simulink model "MinimumJerkPlanner"  (R2024b)
settings: configuration reference "MCConfiguration" (kept outside this file)
undefined symbols (not defined in the file): acc_max, bVelocityMove, InitTrajectory, p0, pos_max, pos_min, target_pos, target_vel, Trajectory_set_pos_end, Trajectory_set_pos_raw, Trajectory_velocity_stop, Ts, vA, vel_max, velAvg, vInvT, vK0, vK1, vK2, vT, vTimer, vV, vX, xA, xInvT, xK0, xK1, xK2, xK3, xStar, xT, xTimer, xV, xX
libraries: simulink x6
settings Model: DataDictionary=MotionController.sldd  Creator=rpumpo  LastModifiedBy=mfussi
settings ConfigSetRef: SourceName=MCConfiguration

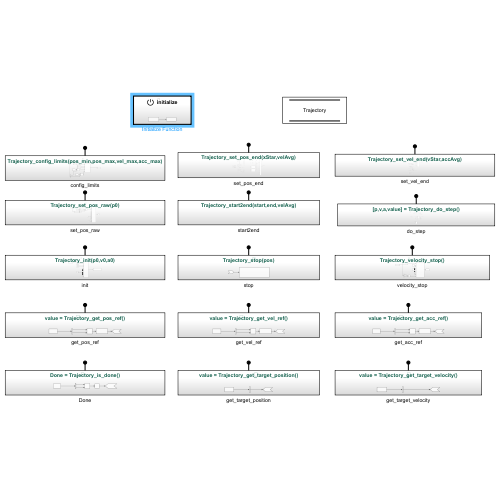
[thumbnail: Simulink's stored preview of the top-level diagram]
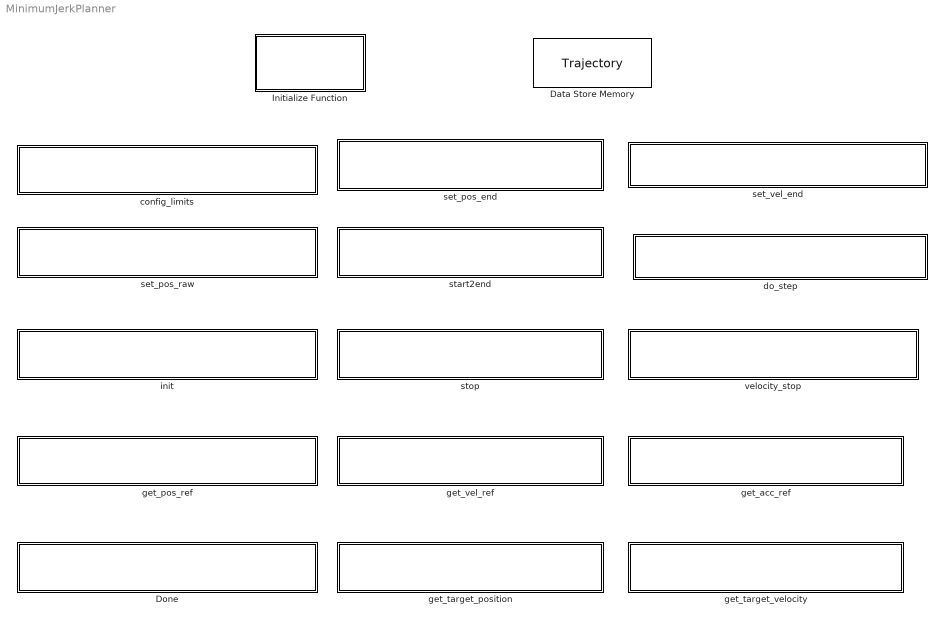
== system MinimumJerkPlanner ==
  Data Store Memory : DataStoreMemory  DataStoreName=Trajectory  WriteAfterWriteMsg=warning  ShowAdditionalParam=off  OutDataTypeStr=Bus: trajectoryhidParameters
  Done : Subsystem  TreatAsAtomicUnit=on
  Initialize Function : Subsystem  TreatAsAtomicUnit=on
  config_limits : Subsystem  TreatAsAtomicUnit=on
  do_step : Subsystem  TreatAsAtomicUnit=on
  get_acc_ref : Subsystem  TreatAsAtomicUnit=on
  get_pos_ref : Subsystem  TreatAsAtomicUnit=on
  get_target_position : Subsystem  TreatAsAtomicUnit=on
  get_target_velocity : Subsystem  TreatAsAtomicUnit=on
  get_vel_ref : Subsystem  TreatAsAtomicUnit=on
  init : Subsystem  TreatAsAtomicUnit=on
  set_pos_end : Subsystem  TreatAsAtomicUnit=on
  set_pos_raw : Subsystem  TreatAsAtomicUnit=on
  set_vel_end : Subsystem  TreatAsAtomicUnit=on
  start2end : Subsystem  TreatAsAtomicUnit=on
  stop : Subsystem  TreatAsAtomicUnit=on
  velocity_stop : Subsystem  TreatAsAtomicUnit=on

== system MinimumJerkPlanner/Done ==
  Trajectory_is_done : TriggerPort  TriggerType=function-call  IsSimulinkFunction=on  FunctionName=Trajectory_is_done  FunctionVisibility=scoped  VariantControl=(inherit)
  Add : Sum  Inputs=+-
  Bus Selector : BusSelector  OutputSignals=xTimer,xT
  Compare To Constant : simulink/Logic and Bit Operations/Compare To Constant  relop=>=  const=0  OutDataTypeStr=boolean
  Data Store Read : DataStoreRead  DataStoreName=Trajectory  IndexOptions=Index vector (dialog)  Indices=1  OutputSizes=1
  Done : ArgOut  OutDataTypeStr=boolean  ArgumentName=Done
  wires:
  Data Store Read/1 -> Bus Selector/1
  Bus Selector/2 -> Add/2  "<xT>"
  Bus Selector/1 -> Add/1  "<xTimer>"
  Add/1 -> Compare To Constant/1
  Compare To Constant/1 -> Done/1

== system MinimumJerkPlanner/Initialize Function ==
  Constant : Constant  Value=InitTrajectory  OutDataTypeStr=Bus: trajectoryhidParameters
  Data Store Write : DataStoreWrite  DataStoreName=Trajectory  IndexOptions=Index vector (dialog)  Indices=1  OutputSizes=1
  Event Listener : EventListener  DisableCoverage=on  EventName=reset
  wires:
  Constant/1 -> Data Store Write/1

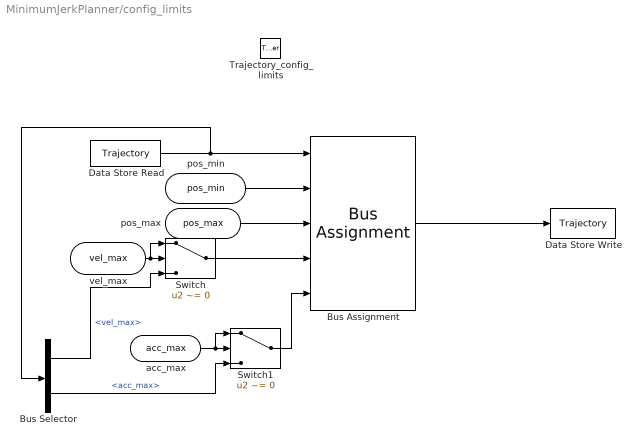
== system MinimumJerkPlanner/config_limits ==
  Trajectory_config_limits : TriggerPort  TriggerType=function-call  IsSimulinkFunction=on  FunctionName=Trajectory_config_limits  FunctionVisibility=scoped  VariantControl=(inherit)
  Bus Assignment : BusAssignment  AssignedSignals=pos_min,pos_max,vel_max,acc_max
  Bus Selector : BusSelector  OutputSignals=vel_max,acc_max
  Data Store Read : DataStoreRead  DataStoreName=Trajectory  IndexOptions=Index vector (dialog)  Indices=1  OutputSizes=1
  Data Store Write : DataStoreWrite  DataStoreName=Trajectory  IndexOptions=Index vector (dialog)  Indices=1  OutputSizes=1
  Switch : Switch  Criteria=u2 ~= 0  SaturateOnIntegerOverflow=off  InputSameDT=off
  Switch1 : Switch  Criteria=u2 ~= 0  SaturateOnIntegerOverflow=off  InputSameDT=off
  pos_min : ArgIn  OutDataTypeStr=single  ArgumentName=pos_min
  pos_max : ArgIn  Port=2  OutDataTypeStr=single  ArgumentName=pos_max
  vel_max : ArgIn  Port=3  OutDataTypeStr=single  ArgumentName=vel_max
  acc_max : ArgIn  Port=4  OutDataTypeStr=single  ArgumentName=acc_max
  wires:
  Data Store Read/1 -> Bus Selector/1, Bus Assignment/1
  pos_min/1 -> Bus Assignment/2
  pos_max/1 -> Bus Assignment/3
  Bus Assignment/1 -> Data Store Write/1
  vel_max/1 -> Switch/1, Switch/2
  Bus Selector/1 -> Switch/3  "<vel_max>"
  Switch/1 -> Bus Assignment/4
  acc_max/1 -> Switch1/1, Switch1/2
  Bus Selector/2 -> Switch1/3  "<acc_max>"
  Switch1/1 -> Bus Assignment/5

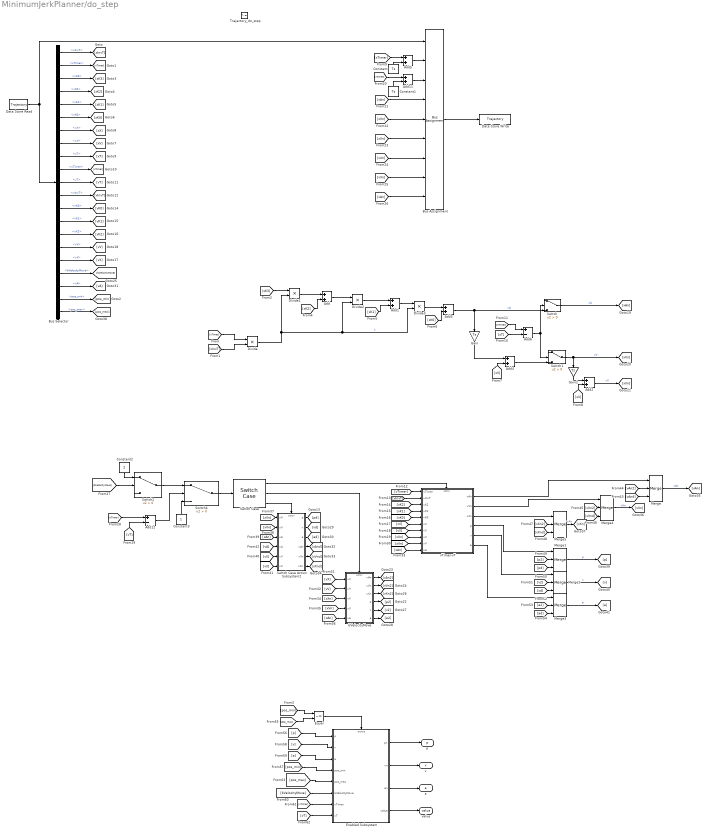
== system MinimumJerkPlanner/do_step ==
  Trajectory_do_step : TriggerPort  TriggerType=function-call  IsSimulinkFunction=on  FunctionName=Trajectory_do_step  FunctionVisibility=scoped  VariantControl=(inherit)
  Add{,1..5,11} (7 alike) : Sum
  Add12 : Sum  Inputs=+-
  Add6 : Sum  Inputs=+-
  Bus Assignment : BusAssignment  AssignedSignals=xTimer,vTimer,xA,xV,xX,vX,vV,vA
  Bus Selector : BusSelector  OutputSignals=xInvT,xTimer,xK3,xK2,xK1,xK0,xX,xV,xT,vTimer,vT,vInvT,vK0,vK1,vK2,vV,vX,bVelocityMove,vA,pos_min,pos_max
  Constant : Constant  Value=Ts  OutDataTypeStr=single
  Constant1 : Constant  Value=Ts  OutDataTypeStr=single
  Constant2 : Constant  Value=2
  Constant3 : Constant
  Data Store Read : DataStoreRead  DataStoreName=Trajectory  IndexOptions=Index vector (dialog)  Indices=1  OutputSizes=1
  Data Store Write : DataStoreWrite  DataStoreName=Trajectory  IndexOptions=Index vector (dialog)  Indices=1  OutputSizes=1
  Divide{,1..3} (4 alike) : Product  Inputs=**
  Enabled Subsystem : Subsystem  TreatAsAtomicUnit=on
  Equal : RelationalOperator  Operator=~=  OutDataTypeStr=boolean  RndMeth=Simplest  InputSameDT=off
  Gain : Gain  Gain=Ts
  Gain2 : Gain  Gain=Ts
  Merge{,1..5} (6 alike) : Merge  Inputs=3
  Switch{,1..2,4} (4 alike) : Switch  Criteria=u2 > Threshold  SaturateOnIntegerOverflow=off  InputSameDT=off
  Switch Case : SwitchCase  CaseConditions={1,2}
  Switch Case Action Subsystem2 : Subsystem  TreatAsAtomicUnit=on
  bVelocityMove : Subsystem  TreatAsAtomicUnit=on
  vTimer-vT : Subsystem  TreatAsAtomicUnit=on
  p : ArgOut  DisableCoverage=on  OutDataTypeStr=single  ArgumentName=p
  v : ArgOut  DisableCoverage=on  Port=2  OutDataTypeStr=single  ArgumentName=v
  a : ArgOut  DisableCoverage=on  Port=3  OutDataTypeStr=single  ArgumentName=a
  value : ArgOut  DisableCoverage=on  Port=4  OutDataTypeStr=int32  ArgumentName=value
  wires:
  Data Store Read/1 -> Bus Assignment/1, Bus Selector/1
  Add4/1 -> Switch1/3
  Add3/1 -> Switch/3, Gain/1  "xA"
  Bus Selector/1 -> [xInvT]  "<xInvT>"
  Bus Selector/2 -> [xTimer]  "<xTimer>"
  [xTimer] -> Divide/1
  [xInvT] -> Divide/2
  Divide/1 -> Divide1/2, Divide2/2, Divide3/2  "t"
  Bus Selector/3 -> [xK3]  "<xK3>"
  Bus Selector/4 -> [xK2]  "<xK2>"
  Bus Selector/5 -> [xK1]  "<xK1>"
  Bus Selector/6 -> [xK0]  "<xK0>"
  [xK3] -> Divide1/1
  Divide1/1 -> Add/1
  [xK2] -> Add/2
  Add/1 -> Divide2/1
  Divide2/1 -> Add1/1
  [xK1] -> Add1/2
  Add1/1 -> Divide3/1
  Divide3/1 -> Add3/1
  [xK0] -> Add3/2
  Bus Selector/7 -> [xX]  "<xX>"
  Bus Selector/8 -> [xV]  "<xV>"
  Gain/1 -> Add4/1
  [xV] -> Add4/2
  Gain2/1 -> Add2/1
  [xX] -> Add2/2
  [xTimer] -> Add5/1
  Constant/1 -> Add5/2
  Add5/1 -> Bus Assignment/2
  Bus Assignment/1 -> Data Store Write/1
  Bus Selector/9 -> [xT]  "<xT>"
  [xTimer] -> Add6/1
  [xT] -> Add6/2
  Add6/1 -> Switch/2, Switch1/2
  Switch1/1 -> Gain2/1, [xVn]  "xV"
  Bus Selector/10 -> [vTimer]  "<vTimer>"
  Bus Selector/11 -> [vT]  "<vT>"
  Bus Selector/12 -> [vInvT]  "<vInvT>"
  Bus Selector/13 -> [vK0]  "<vK0>"
  Bus Selector/14 -> [vK1]  "<vK1>"
  Bus Selector/15 -> [vK2]  "<vK2>"
  Bus Selector/16 -> [vV]  "<vV>"
  Bus Selector/17 -> [vX]  "<vX>"
  Switch/1 -> [xAn]  "xA"
  Add2/1 -> [xXn]  "xX"
  [xAn] -> Bus Assignment/4
  [xVn] -> Bus Assignment/5
  [xXn] -> Bus Assignment/6
  [vXn] -> Bus Assignment/7
  [vVn] -> Bus Assignment/8
  [vAn] -> Bus Assignment/9
  Bus Selector/18 -> [bVelocityMove]  "<bVelocityMove>"
  [bVelocityMove] -> Switch2/2
  Constant2/1 -> Switch2/1
  Switch Case/1 -> vTimer-vT/Action
  Switch Case/2 -> bVelocityMove/Action
  Switch2/1 -> Switch4/1
  [vX] -> bVelocityMove/1(vX)
  [vV] -> bVelocityMove/2(vV)
  [vTimer] -> Add12/1
  [vT] -> Add12/2
  Add12/1 -> Switch4/2
  Constant3/1 -> Switch4/3
  Switch4/1 -> Switch Case/1
  [vTimer] -> vTimer-vT/1(vTimer)
  [vInvT] -> vTimer-vT/2(vInvT)
  [vK2] -> vTimer-vT/3(vK2)
  [vK1] -> vTimer-vT/4(vK1)
  [vK0] -> vTimer-vT/5(vK0)
  [vV] -> vTimer-vT/6(vV)
  [vX] -> vTimer-vT/7(vX)
  [vTimer] -> Add11/1
  Constant1/1 -> Add11/2
  Add11/1 -> Bus Assignment/3
  [xXn] -> vTimer-vT/8(xX)
  [xVn] -> vTimer-vT/9(xV)
  [xAn] -> vTimer-vT/10(xA)
  [xXn] -> bVelocityMove/3(xX)
  [xVn] -> bVelocityMove/4(xV)
  [xAn] -> bVelocityMove/5(xA)
  Switch Case/3 -> Switch Case Action Subsystem2/Action
  [xXn] -> Switch Case Action Subsystem2/1(xX)
  [xVn] -> Switch Case Action Subsystem2/2(xV)
  [xAn] -> Switch Case Action Subsystem2/3(xA)
  Merge/1 -> [vAn]  "vAn"
  Merge1/1 -> [p]  "p"
  [vV] -> Switch Case Action Subsystem2/5(vV)
  [vX] -> Switch Case Action Subsystem2/6(vX)
  [vA] -> Switch Case Action Subsystem2/4(vA)
  Switch Case Action Subsystem2/1(p) -> [pd]
  bVelocityMove/4(p) -> [p2]
  vTimer-vT/4(p) -> Merge1/1
  vTimer-vT/5(v) -> Merge2/1
  vTimer-vT/6(a) -> Merge3/1
  bVelocityMove/6(a) -> [a2]
  bVelocityMove/5(v) -> [v2]
  Switch Case Action Subsystem2/2(v) -> [vd]
  Switch Case Action Subsystem2/3(a) -> [ad]
  Bus Selector/19 -> [vA]  "<vA>"
  vTimer-vT/1(vAn) -> Merge/1
  [vAnd] -> Merge/3
  [vAn2] -> Merge/2
  bVelocityMove/1(vAn) -> [vAn2]
  bVelocityMove/2(vVn) -> [vVn2]
  bVelocityMove/3(vXn) -> [vXn2]
  Switch Case Action Subsystem2/4(vAn) -> [vAnd]
  Switch Case Action Subsystem2/5(vVn) -> [vVnd]
  Switch Case Action Subsystem2/6(vXn) -> [vXnd]
  vTimer-vT/2(vVn) -> Merge4/1
  [vVn2] -> Merge4/2
  [vVnd] -> Merge4/3
  Merge4/1 -> [vVn]  "vVn"
  vTimer-vT/3(vXn) -> Merge5/1
  Merge5/1 -> [vXn]  "vXn"
  [vXn2] -> Merge5/2
  [vXnd] -> Merge5/3
  [p2] -> Merge1/2
  [pd] -> Merge1/3
  [v2] -> Merge2/2
  [vd] -> Merge2/3
  [a2] -> Merge3/2
  [ad] -> Merge3/3
  Bus Selector/20 -> [pos_min]  "<pos_min>"
  Bus Selector/21 -> [pos_max]  "<pos_max>"
  [pos_min] -> Equal/1
  [pos_max] -> Equal/2
  Equal/1 -> Enabled Subsystem/Enable
  [p] -> Enabled Subsystem/1(p)
  [pos_min] -> Enabled Subsystem/4(pos_min)
  Merge2/1 -> [v]  "v"
  Merge3/1 -> [a]  "a"
  [v] -> Enabled Subsystem/2(v)
  [a] -> Enabled Subsystem/3(a)
  [bVelocityMove] -> Enabled Subsystem/6(bVelocityMove)
  [vTimer] -> Enabled Subsystem/7(vTimer)
  [vT] -> Enabled Subsystem/8(vT)
  [pos_max] -> Enabled Subsystem/5(pos_max)
  Enabled Subsystem/2(vn) -> v/1
  Enabled Subsystem/3(an) -> a/1
  Enabled Subsystem/1(pn) -> p/1
  Enabled Subsystem/4(value) -> value/1

== system MinimumJerkPlanner/get_acc_ref ==
  Trajectory_get_acc_ref : TriggerPort  TriggerType=function-call  IsSimulinkFunction=on  FunctionName=Trajectory_get_acc_ref  FunctionVisibility=scoped  VariantControl=(inherit)
  Add : Sum
  Bus Selector : BusSelector  OutputSignals=xA,vA
  Data Store Read : DataStoreRead  DataStoreName=Trajectory  IndexOptions=Index vector (dialog)  Indices=1  OutputSizes=1
  Data Type Conversion : DataTypeConversion  OutDataTypeStr=int32  SaturateOnIntegerOverflow=off  RndMeth=Floor
  value : ArgOut  OutDataTypeStr=int32  ArgumentName=value
  wires:
  Data Store Read/1 -> Bus Selector/1
  Add/1 -> Data Type Conversion/1
  Data Type Conversion/1 -> value/1
  Bus Selector/1 -> Add/1  "<xA>"
  Bus Selector/2 -> Add/2  "<vA>"

== system MinimumJerkPlanner/get_pos_ref ==
  Trajectory_get_pos_ref : TriggerPort  TriggerType=function-call  IsSimulinkFunction=on  FunctionName=Trajectory_get_pos_ref  FunctionVisibility=scoped  VariantControl=(inherit)
  Add : Sum
  Bus Selector : BusSelector  OutputSignals=xX,vX
  Data Store Read : DataStoreRead  DataStoreName=Trajectory  IndexOptions=Index vector (dialog)  Indices=1  OutputSizes=1
  Data Type Conversion : DataTypeConversion  OutDataTypeStr=int32  SaturateOnIntegerOverflow=off  RndMeth=Floor
  value : ArgOut  OutDataTypeStr=int32  ArgumentName=value
  wires:
  Data Store Read/1 -> Bus Selector/1
  Bus Selector/1 -> Add/1  "<xX>"
  Bus Selector/2 -> Add/2  "<vX>"
  Add/1 -> Data Type Conversion/1
  Data Type Conversion/1 -> value/1

== system MinimumJerkPlanner/get_target_position ==
  Trajectory_get_target_position : TriggerPort  TriggerType=function-call  IsSimulinkFunction=on  FunctionName=Trajectory_get_target_position  FunctionVisibility=scoped  VariantControl=(inherit)
  Bus Selector : BusSelector  OutputSignals=target_pos
  Data Store Read : DataStoreRead  DataStoreName=Trajectory  IndexOptions=Index vector (dialog)  Indices=1  OutputSizes=1
  value : ArgOut  OutDataTypeStr=single  ArgumentName=value
  wires:
  Data Store Read/1 -> Bus Selector/1
  Bus Selector/1 -> value/1  "<target_pos>"

== system MinimumJerkPlanner/get_target_velocity ==
  Trajectory_get_target_velocity : TriggerPort  TriggerType=function-call  IsSimulinkFunction=on  FunctionName=Trajectory_get_target_velocity  FunctionVisibility=scoped  VariantControl=(inherit)
  Bus Selector : BusSelector  OutputSignals=target_vel
  Data Store Read : DataStoreRead  DataStoreName=Trajectory  IndexOptions=Index vector (dialog)  Indices=1  OutputSizes=1
  value : ArgOut  OutDataTypeStr=single  ArgumentName=value
  wires:
  Data Store Read/1 -> Bus Selector/1
  Bus Selector/1 -> value/1  "<target_vel>"

== system MinimumJerkPlanner/get_vel_ref ==
  Trajectory_get_vel_ref : TriggerPort  TriggerType=function-call  IsSimulinkFunction=on  FunctionName=Trajectory_get_vel_ref  FunctionVisibility=scoped  VariantControl=(inherit)
  Add : Sum
  Bus Selector : BusSelector  OutputSignals=xV,vV
  Data Store Read : DataStoreRead  DataStoreName=Trajectory  IndexOptions=Index vector (dialog)  Indices=1  OutputSizes=1
  Data Type Conversion : DataTypeConversion  OutDataTypeStr=int32  SaturateOnIntegerOverflow=off  RndMeth=Floor
  value : ArgOut  OutDataTypeStr=int32  ArgumentName=value
  wires:
  Data Store Read/1 -> Bus Selector/1
  Add/1 -> Data Type Conversion/1
  Data Type Conversion/1 -> value/1
  Bus Selector/1 -> Add/1  "<xV>"
  Bus Selector/2 -> Add/2  "<vV>"

== system MinimumJerkPlanner/init ==
  Trajectory_init : TriggerPort  TriggerType=function-call  IsSimulinkFunction=on  FunctionName=Trajectory_init  FunctionVisibility=scoped  VariantControl=(inherit)
  Bus Assignment : BusAssignment  AssignedSignals=xX,xV,xA,xTimer,xT,vX,vV,vA,vTimer,vT
  Constant : Constant  Value=0  OutDataTypeStr=single
  Data Store Read : DataStoreRead  DataStoreName=Trajectory  IndexOptions=Index vector (dialog)  Indices=1  OutputSizes=1
  Data Store Write : DataStoreWrite  DataStoreName=Trajectory  IndexOptions=Index vector (dialog)  Indices=1  OutputSizes=1
  p0 : ArgIn  OutDataTypeStr=single  ArgumentName=p0
  v0 : ArgIn  Port=2  OutDataTypeStr=single  ArgumentName=v0
  a0 : ArgIn  Port=3  OutDataTypeStr=single  ArgumentName=a0
  wires:
  Data Store Read/1 -> Bus Assignment/1
  p0/1 -> Bus Assignment/2
  v0/1 -> Bus Assignment/3
  a0/1 -> Bus Assignment/4
  Constant/1 -> Bus Assignment/10, Bus Assignment/11, Bus Assignment/9, Bus Assignment/5, Bus Assignment/6, Bus Assignment/7, Bus Assignment/8
  Bus Assignment/1 -> Data Store Write/1

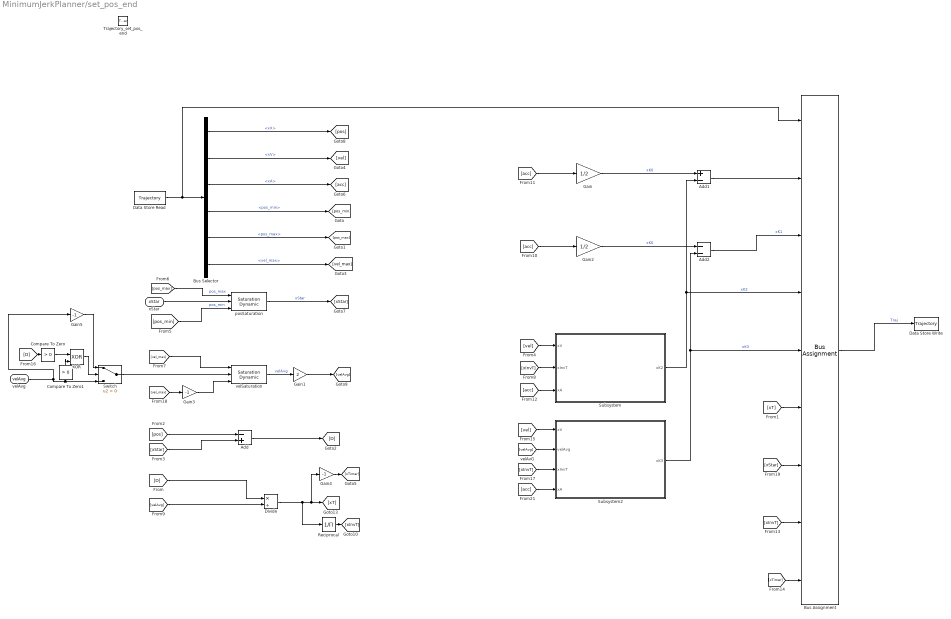
== system MinimumJerkPlanner/set_pos_end ==
  Trajectory_set_pos_end : TriggerPort  TriggerType=function-call  IsSimulinkFunction=on  FunctionName=Trajectory_set_pos_end  FunctionVisibility=scoped  VariantControl=(inherit)
  Add : Sum  Inputs=-+
  Add1 : Sum  Inputs=+-
  Add2 : Sum  Inputs=--
  Bus Assignment : BusAssignment  AssignedSignals=xK0,xK1,xK2,xK3,xT,target_pos,xInvT,xTimer
  Bus Selector : BusSelector  OutputSignals=xX,xV,xA,pos_min,pos_max,vel_max
  Compare To Zero : simulink/Logic and Bit Operations/Compare To Zero  relop=>  OutDataTypeStr=boolean
  Compare To Zero1 : simulink/Logic and Bit Operations/Compare To Zero  relop=>  OutDataTypeStr=boolean
  Data Store Read : DataStoreRead  DataStoreName=Trajectory  IndexOptions=Index vector (dialog)  Indices=1  OutputSizes=1
  Data Store Write : DataStoreWrite  DataStoreName=Trajectory  IndexOptions=Index vector (dialog)  Indices=1  OutputSizes=1
  Divide : Product  Inputs=*/
  Gain : Gain  Gain=1/2
  Gain1 : Gain  Gain=2
  Gain2 : Gain  Gain=1/2
  Gain3 : Gain  Gain=-1
  Gain4 : Gain  Gain=-1
  Gain5 : Gain  Gain=-1
  Reciprocal : Product  Inputs=/
  Subsystem : Subsystem
  Subsystem2 : Subsystem
  Switch : Switch  Criteria=u2 > Threshold  SaturateOnIntegerOverflow=off  InputSameDT=off
  XOR : Logic  Operator=XOR  IconShape=distinctive  AllPortsSameDT=off  OutDataTypeStr=boolean
  posSaturation : simulink/Discontinuities/Saturation Dynamic  OutMin=[]  OutMax=[]  OutDataTypeStr=Inherit: Same as second input  OutDataType=fixdt(1, 16)  OutScaling=2^-10  DoSatur=off
  velSaturation : simulink/Discontinuities/Saturation Dynamic  OutMin=[]  OutMax=[]  OutDataTypeStr=Inherit: Same as second input  OutDataType=fixdt(1, 16)  OutScaling=2^-10  DoSatur=off
  xStar : ArgIn  DisableCoverage=on  OutDataTypeStr=single  ArgumentName=xStar
  velAvg : ArgIn  DisableCoverage=on  Port=2  OutDataTypeStr=single  ArgumentName=velAvg
  wires:
  Subsystem/1(xK2) -> Add1/2, Bus Assignment/4  "xK2"
  [vel_max] -> Gain3/1
  [vel_max] -> velSaturation/1
  [pos] -> Add/1
  Divide/1 -> Reciprocal/1, Gain4/1, [xT]
  Bus Selector/6 -> [vel_max]  "<vel_max>"
  Gain3/1 -> velSaturation/3
  Add2/1 -> Bus Assignment/3  "xK1"
  Add/1 -> [D]
  [xStar] -> Add/2
  [pos_min] -> posSaturation/3  "pos_min"
  xStar/1 -> posSaturation/2
  [D] -> Divide/1
  [pos_max] -> posSaturation/1  "pos_max"
  Bus Selector/4 -> [pos_min]  "<pos_min>"
  Bus Selector/2 -> [vel]  "<xV>"
  Subsystem2/1(xK3) -> Add2/2, Bus Assignment/5  "xK3"
  [xT] -> Bus Assignment/6
  Data Store Read/1 -> Bus Assignment/1, Bus Selector/1
  Bus Selector/3 -> [acc]  "<xA>"
  [xStar] -> Bus Assignment/7
  [velAvg] -> Divide/2
  Bus Assignment/1 -> Data Store Write/1  "Traj"
  posSaturation/1 -> [xStar]  "xStar"
  [acc] -> Gain/1
  Bus Selector/1 -> [pos]  "<xX>"
  Bus Selector/5 -> [pos_max]  "<pos_max>"
  velSaturation/1 -> Gain1/1  "velAvg"
  [vel] -> Subsystem/1(xV)
  Reciprocal/1 -> [xInvT]
  [xInvT] -> Subsystem/2(xInvT)
  [acc] -> Subsystem/3(xA)
  [vel] -> Subsystem2/1(xV)
  [velAvg] -> Subsystem2/2(velAvg)
  [xInvT] -> Subsystem2/3(xInvT)
  [acc] -> Subsystem2/4(xA)
  Gain/1 -> Add1/1  "xK0"
  Add1/1 -> Bus Assignment/2
  [acc] -> Gain2/1
  Gain2/1 -> Add2/1  "xK0"
  Gain1/1 -> [velAvg]
  [xInvT] -> Bus Assignment/8
  Gain4/1 -> [xTimer]
  [xTimer] -> Bus Assignment/9
  [D] -> Compare To Zero/1
  velAvg/1 -> Switch/3, Compare To Zero1/1, Gain5/1
  XOR/1 -> Switch/2
  Gain5/1 -> Switch/1
  Switch/1 -> velSaturation/2
  Compare To Zero/1 -> XOR/1
  Compare To Zero1/1 -> XOR/2

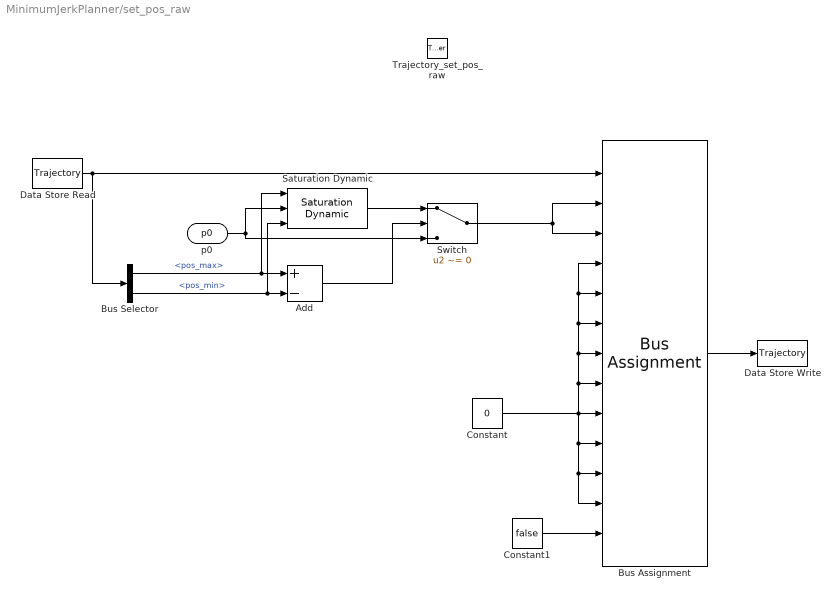
== system MinimumJerkPlanner/set_pos_raw ==
  Trajectory_set_pos_raw : TriggerPort  TriggerType=function-call  IsSimulinkFunction=on  FunctionName=Trajectory_set_pos_raw  FunctionVisibility=scoped  VariantControl=(inherit)
  Add : Sum  Inputs=+-
  Bus Assignment : BusAssignment  AssignedSignals=target_pos,xX,xV,xA,xTimer,xT,vX,vV,vA,vTimer,vT,bVelocityMove
  Bus Selector : BusSelector  OutputSignals=pos_max,pos_min
  Constant : Constant  Value=0  OutDataTypeStr=single
  Constant1 : Constant  Value=false  OutDataTypeStr=boolean
  Data Store Read : DataStoreRead  DataStoreName=Trajectory  IndexOptions=Index vector (dialog)  Indices=1  OutputSizes=1
  Data Store Write : DataStoreWrite  DataStoreName=Trajectory  IndexOptions=Index vector (dialog)  Indices=1  OutputSizes=1
  Saturation Dynamic : simulink/Discontinuities/Saturation Dynamic  OutMin=[]  OutMax=[]  OutDataTypeStr=Inherit: Same as second input  OutDataType=fixdt(1, 16)  OutScaling=2^-10  DoSatur=off
  Switch : Switch  Criteria=u2 ~= 0  SaturateOnIntegerOverflow=off  InputSameDT=off
  p0 : ArgIn  OutDataTypeStr=single  ArgumentName=p0
  wires:
  Bus Assignment/1 -> Data Store Write/1
  Data Store Read/1 -> Bus Assignment/1, Bus Selector/1
  Add/1 -> Switch/2
  Saturation Dynamic/1 -> Switch/1
  p0/1 -> Switch/3, Saturation Dynamic/2
  Switch/1 -> Bus Assignment/2, Bus Assignment/3
  Bus Selector/2 -> Saturation Dynamic/3, Add/2  "<pos_min>"
  Bus Selector/1 -> Saturation Dynamic/1, Add/1  "<pos_max>"
  Constant/1 -> Bus Assignment/5, Bus Assignment/4, Bus Assignment/6, Bus Assignment/7, Bus Assignment/8, Bus Assignment/10, Bus Assignment/11, Bus Assignment/12, Bus Assignment/9
  Constant1/1 -> Bus Assignment/13

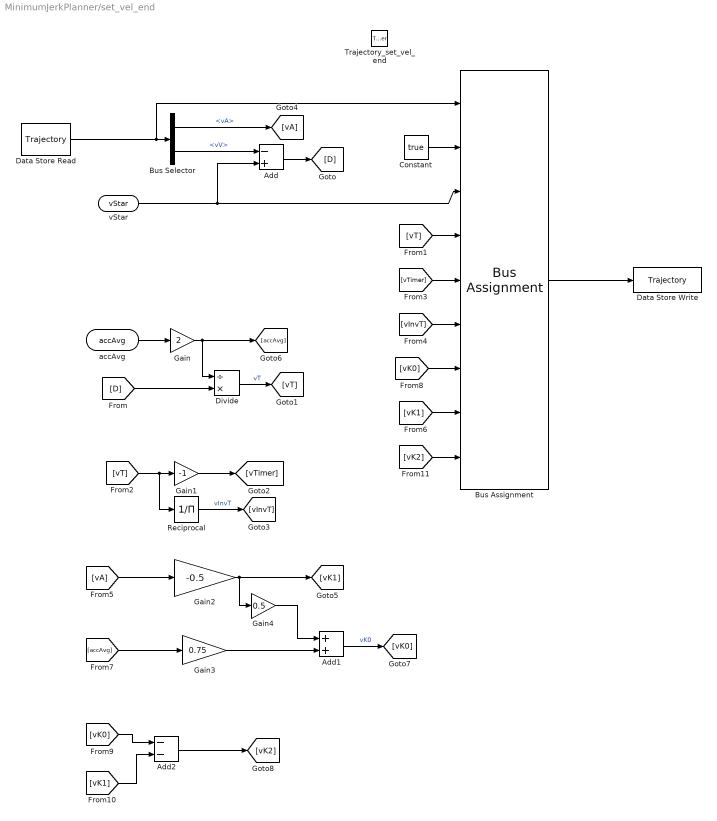
== system MinimumJerkPlanner/set_vel_end ==
  Trajectory_set_vel_end : TriggerPort  TriggerType=function-call  IsSimulinkFunction=on  FunctionName=Trajectory_set_vel_end  FunctionVisibility=scoped  VariantControl=(inherit)
  Add : Sum  Inputs=-+
  Add1 : Sum
  Add2 : Sum  Inputs=--
  Bus Assignment : BusAssignment  AssignedSignals=bVelocityMove,target_vel,vT,vTimer,vInvT,vK0,vK1,vK2
  Bus Selector : BusSelector  OutputSignals=vA,vV
  Constant : Constant  Value=true  OutDataTypeStr=boolean
  Data Store Read : DataStoreRead  DataStoreName=Trajectory  IndexOptions=Index vector (dialog)  Indices=1  OutputSizes=1
  Data Store Write : DataStoreWrite  DataStoreName=Trajectory  IndexOptions=Index vector (dialog)  Indices=1  OutputSizes=1
  Divide : Product  Inputs=/*
  Gain : Gain  Gain=2
  Gain1 : Gain  Gain=-1
  Gain2 : Gain  Gain=-0.5
  Gain3 : Gain  Gain=0.75
  Gain4 : Gain  Gain=0.5
  Reciprocal : Product  Inputs=/
  vStar : ArgIn  OutDataTypeStr=single  ArgumentName=vStar
  accAvg : ArgIn  Port=2  OutDataTypeStr=single  ArgumentName=accAvg
  wires:
  Data Store Read/1 -> Bus Assignment/1, Bus Selector/1
  Bus Assignment/1 -> Data Store Write/1
  Constant/1 -> Bus Assignment/2
  vStar/1 -> Add/2, Bus Assignment/3
  Bus Selector/2 -> Add/1  "<vV>"
  Add/1 -> [D]
  accAvg/1 -> Gain/1
  [D] -> Divide/2
  Gain/1 -> [accAvg], Divide/1
  Divide/1 -> [vT]  "vT"
  [vT] -> Bus Assignment/4
  [vT] -> Reciprocal/1, Gain1/1
  Gain1/1 -> [vTimer]
  [vTimer] -> Bus Assignment/5
  Reciprocal/1 -> [vInvT]  "vInvT"
  [vInvT] -> Bus Assignment/6
  Bus Selector/1 -> [vA]  "<vA>"
  [vA] -> Gain2/1
  Gain2/1 -> Gain4/1, [vK1]
  [vK1] -> Bus Assignment/8
  [accAvg] -> Gain3/1
  Gain3/1 -> Add1/2
  Gain4/1 -> Add1/1
  Add1/1 -> [vK0]  "vK0"
  [vK0] -> Bus Assignment/7
  [vK0] -> Add2/1
  [vK1] -> Add2/2
  Add2/1 -> [vK2]
  [vK2] -> Bus Assignment/9

== system MinimumJerkPlanner/start2end ==
  Trajectory_start2end : TriggerPort  TriggerType=function-call  IsSimulinkFunction=on  FunctionName=Trajectory_start2end  FunctionVisibility=scoped  VariantControl=(inherit)
  Function Caller : FunctionCaller  FunctionPrototype=Trajectory_set_pos_raw(p0)  InputArgumentSpecifications=<Enter example>  OutputArgumentSpecifications=<Enter example>
  Function Caller2 : FunctionCaller  FunctionPrototype=Trajectory_set_pos_end(xStar,velAvg)  InputArgumentSpecifications=<Enter example>  OutputArgumentSpecifications=<Enter example>
  start : ArgIn  OutDataTypeStr=single  ArgumentName=start
  end : ArgIn  Port=2  OutDataTypeStr=single  ArgumentName=end
  velAvg : ArgIn  Port=3  OutDataTypeStr=single  ArgumentName=velAvg
  wires:
  start/1 -> Function Caller/1
  end/1 -> Function Caller2/1
  velAvg/1 -> Function Caller2/2

== system MinimumJerkPlanner/stop ==
  Trajectory_stop : TriggerPort  TriggerType=function-call  IsSimulinkFunction=on  FunctionName=Trajectory_stop  FunctionVisibility=scoped  VariantControl=(inherit)
  Function Caller4 : FunctionCaller  FunctionPrototype=Trajectory_set_pos_raw(p0)  InputArgumentSpecifications=<Enter example>  OutputArgumentSpecifications=<Enter example>
  pos : ArgIn  OutDataTypeStr=single  ArgumentName=pos
  wires:
  pos/1 -> Function Caller4/1

== system MinimumJerkPlanner/velocity_stop ==
  Trajectory_velocity_stop : TriggerPort  TriggerType=function-call  IsSimulinkFunction=on  FunctionName=Trajectory_velocity_stop  FunctionVisibility=scoped  VariantControl=(inherit)
  Add : Sum
  Bus Assignment : BusAssignment  AssignedSignals=bVelocityMove,vTimer,vT,vX,vV,vA,target_vel,xX
  Bus Selector : BusSelector  OutputSignals=xX,vX
  Data Store Read : DataStoreRead  DataStoreName=Trajectory  IndexOptions=Index vector (dialog)  Indices=1  OutputSizes=1
  Data Store Write : DataStoreWrite  DataStoreName=Trajectory  IndexOptions=Index vector (dialog)  Indices=1  OutputSizes=1
  Zero : Constant  Value=false  OutDataTypeStr=boolean
  Zero1 : Constant  Value=0  OutDataTypeStr=single
  wires:
  Bus Assignment/1 -> Data Store Write/1
  Data Store Read/1 -> Bus Assignment/1, Bus Selector/1
  Zero/1 -> Bus Assignment/2
  Zero1/1 -> Bus Assignment/8, Bus Assignment/7, Bus Assignment/6, Bus Assignment/4, Bus Assignment/3, Bus Assignment/5
  Bus Selector/2 -> Add/2  "<vX>"
  Bus Selector/1 -> Add/1  "<xX>"
  Add/1 -> Bus Assignment/9

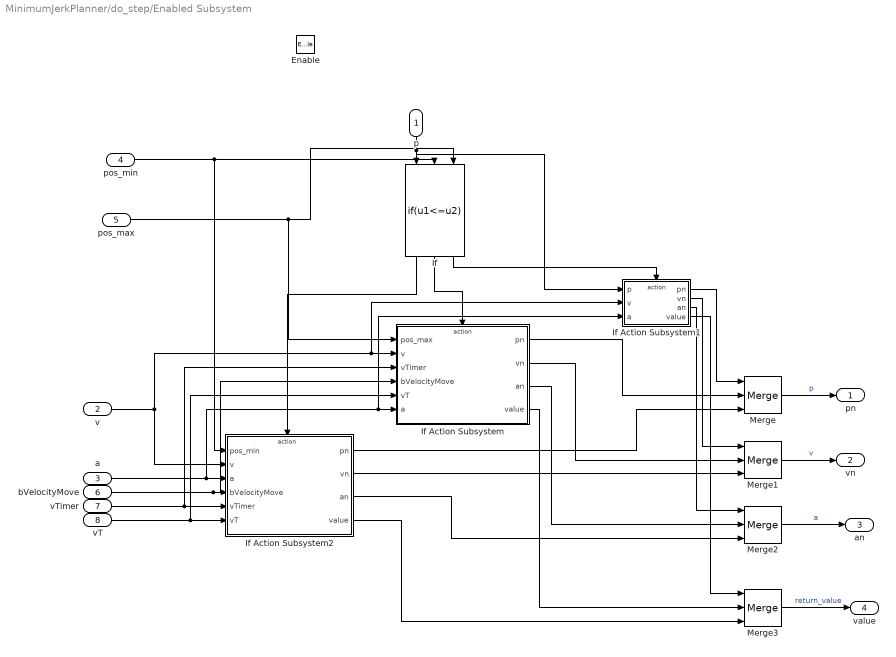
== system MinimumJerkPlanner/do_step/Enabled Subsystem ==
  p : Inport
  v : Inport  Port=2
  a : Inport  Port=3
  pos_min : Inport  Port=4
  pos_max : Inport  Port=5
  bVelocityMove : Inport  Port=6
  vTimer : Inport  Port=7
  vT : Inport  Port=8
  Enable : EnablePort
  If : If  NumInputs=3  IfExpression=u1<=u2  ElseIfExpressions=u1>=u3
  If Action Subsystem : Subsystem  TreatAsAtomicUnit=on
  If Action Subsystem1 : Subsystem  TreatAsAtomicUnit=on
  If Action Subsystem2 : Subsystem  TreatAsAtomicUnit=on
  Merge{,1..3} (4 alike) : Merge  Inputs=3
  pn : Outport
  vn : Outport  Port=2
  an : Outport  Port=3
  value : Outport  Port=4  OutDataTypeStr=int32
  wires:
  pos_min/1 -> If Action Subsystem2/1(pos_min), If/2
  p/1 -> If Action Subsystem1/1(p), If/1
  v/1 -> If Action Subsystem1/2(v), If Action Subsystem/2(v), If Action Subsystem2/2(v)
  bVelocityMove/1 -> If Action Subsystem/4(bVelocityMove), If Action Subsystem2/4(bVelocityMove)
  vTimer/1 -> If Action Subsystem2/5(vTimer), If Action Subsystem/3(vTimer)
  vT/1 -> If Action Subsystem/5(vT), If Action Subsystem2/6(vT)
  a/1 -> If Action Subsystem1/3(a), If Action Subsystem/6(a), If Action Subsystem2/3(a)
  If/1 -> If Action Subsystem2/Action
  If/2 -> If Action Subsystem/Action
  pos_max/1 -> If Action Subsystem/1(pos_max), If/3
  If/3 -> If Action Subsystem1/Action
  If Action Subsystem1/1(pn) -> Merge/1
  If Action Subsystem/1(pn) -> Merge/2
  If Action Subsystem2/1(pn) -> Merge/3
  Merge/1 -> pn/1  "p"
  Merge1/1 -> vn/1  "v"
  If Action Subsystem1/2(vn) -> Merge1/1
  If Action Subsystem/2(vn) -> Merge1/2
  If Action Subsystem2/2(vn) -> Merge1/3
  If Action Subsystem1/3(an) -> Merge2/1
  If Action Subsystem/3(an) -> Merge2/2
  If Action Subsystem2/3(an) -> Merge2/3
  Merge2/1 -> an/1  "a"
  Merge3/1 -> value/1  "return_value"
  If Action Subsystem1/4(value) -> Merge3/1
  If Action Subsystem/4(value) -> Merge3/2
  If Action Subsystem2/4(value) -> Merge3/3

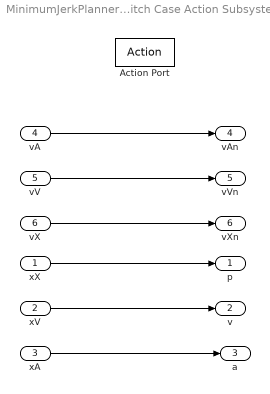
== system MinimumJerkPlanner/do_step/Switch Case Action Subsystem2 ==
  xX : Inport
  xV : Inport  Port=2
  xA : Inport  Port=3
  vA : Inport  Port=4
  vV : Inport  Port=5
  vX : Inport  Port=6
  Action Port : ActionPort  ActionPortLabel=default:
  p : Outport
  v : Outport  Port=2
  a : Outport  Port=3
  vAn : Outport  Port=4
  vVn : Outport  Port=5
  vXn : Outport  Port=6
  wires:
  xX/1 -> p/1
  xV/1 -> v/1
  xA/1 -> a/1
  vA/1 -> vAn/1
  vV/1 -> vVn/1
  vX/1 -> vXn/1

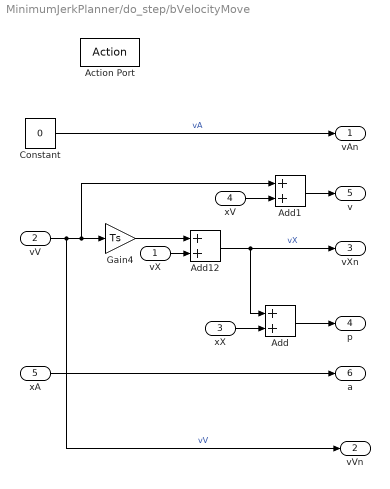
== system MinimumJerkPlanner/do_step/bVelocityMove ==
  vX : Inport
  vV : Inport  Port=2
  xX : Inport  Port=3
  xV : Inport  Port=4
  xA : Inport  Port=5
  Action Port : ActionPort  ActionPortLabel=case [ 2 ]:
  Add : Sum
  Add1 : Sum
  Add12 : Sum
  Constant : Constant  Value=0  OutDataTypeStr=single
  Gain4 : Gain  Gain=Ts
  vAn : Outport
  vVn : Outport  Port=2
  vXn : Outport  Port=3
  p : Outport  Port=4
  v : Outport  Port=5
  a : Outport  Port=6
  wires:
  vX/1 -> Add12/2
  Gain4/1 -> Add12/1
  Add12/1 -> Add/1, vXn/1  "vX"
  vV/1 -> vVn/1, Add1/1, Gain4/1  "vV"
  xA/1 -> a/1
  Constant/1 -> vAn/1  "vA"
  xV/1 -> Add1/2
  Add/1 -> p/1
  xX/1 -> Add/2
  Add1/1 -> v/1

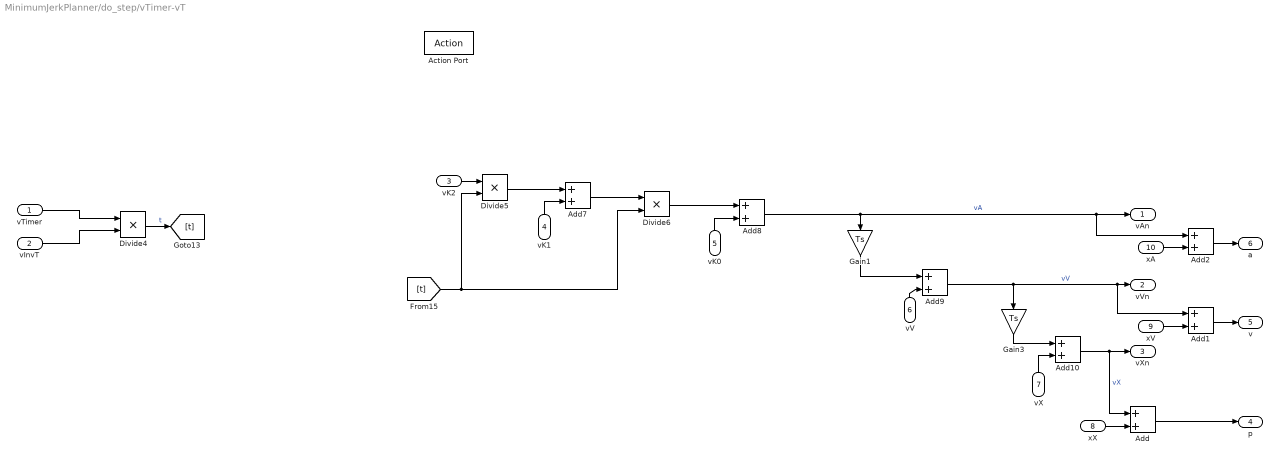
== system MinimumJerkPlanner/do_step/vTimer-vT ==
  vTimer : Inport
  vInvT : Inport  Port=2
  vK2 : Inport  Port=3
  vK1 : Inport  Port=4
  vK0 : Inport  Port=5
  vV : Inport  Port=6
  vX : Inport  Port=7
  xX : Inport  Port=8
  xV : Inport  Port=9
  xA : Inport  Port=10
  Action Port : ActionPort  ActionPortLabel=case [ 1 ]:
  Add{,1..2,7..10} (7 alike) : Sum
  Divide4 : Product  Inputs=**
  Divide5 : Product  Inputs=**
  Divide6 : Product  Inputs=**
  Gain1 : Gain  Gain=Ts
  Gain3 : Gain  Gain=Ts
  vAn : Outport
  vVn : Outport  Port=2
  vXn : Outport  Port=3
  p : Outport  Port=4
  v : Outport  Port=5
  a : Outport  Port=6
  wires:
  Add8/1 -> Add2/1, vAn/1, Gain1/1  "vA"
  vX/1 -> Add10/2
  Divide4/1 -> [t]  "t"
  vTimer/1 -> Divide4/1
  vInvT/1 -> Divide4/2
  vK1/1 -> Add7/2
  Add7/1 -> Divide6/1
  Add10/1 -> Add/1, vXn/1  "vX"
  vK2/1 -> Divide5/1
  Divide6/1 -> Add8/1
  [t] -> Divide5/2, Divide6/2
  Divide5/1 -> Add7/1
  vK0/1 -> Add8/2
  Gain3/1 -> Add10/1
  Add9/1 -> Add1/1, vVn/1, Gain3/1  "vV"
  Gain1/1 -> Add9/1
  vV/1 -> Add9/2
  xX/1 -> Add/2
  Add/1 -> p/1
  xV/1 -> Add1/2
  Add1/1 -> v/1
  Add2/1 -> a/1
  xA/1 -> Add2/2

== system MinimumJerkPlanner/set_pos_end/Subsystem ==
  xV : Inport
  xInvT : Inport  Port=2
  xA : Inport  Port=3
  Add : Sum
  Divide : Product  Inputs=**
  Gain : Gain  Gain=0.75
  xK2 : Outport
  wires:
  xA/1 -> Add/1
  xV/1 -> Divide/1
  xInvT/1 -> Divide/2
  Divide/1 -> Add/2
  Add/1 -> Gain/1
  Gain/1 -> xK2/1

== system MinimumJerkPlanner/set_pos_end/Subsystem2 ==
  xV : Inport
  velAvg : Inport  Port=2
  xInvT : Inport  Port=3
  xA : Inport  Port=4
  Add : Sum  Inputs=+-
  Add1 : Sum  Inputs=--
  Divide : Product  Inputs=**
  Gain : Gain  Gain=3.75
  Gain1 : Gain  Gain=1.25
  xK3 : Outport
  wires:
  xV/1 -> Add/1
  velAvg/1 -> Add/2
  Add/1 -> Divide/1
  xInvT/1 -> Divide/2
  Divide/1 -> Gain/1
  Gain/1 -> Add1/1
  xA/1 -> Gain1/1
  Gain1/1 -> Add1/2
  Add1/1 -> xK3/1

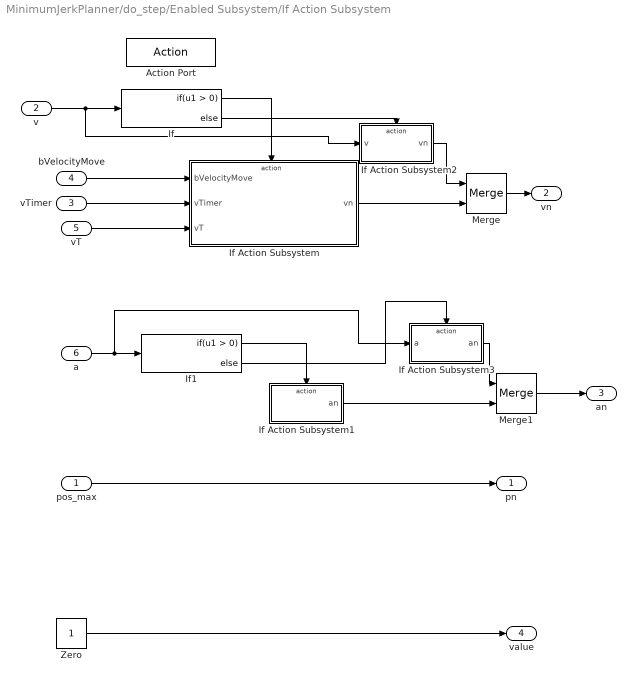
== system MinimumJerkPlanner/do_step/Enabled Subsystem/If Action Subsystem ==
  pos_max : Inport
  v : Inport  Port=2
  vTimer : Inport  Port=3
  bVelocityMove : Inport  Port=4
  vT : Inport  Port=5
  a : Inport  Port=6
  Action Port : ActionPort  ActionPortLabel=elseif(u1>=u3)
  If : If
  If Action Subsystem : Subsystem  TreatAsAtomicUnit=on
  If Action Subsystem1 : Subsystem  TreatAsAtomicUnit=on
  If Action Subsystem2 : Subsystem  TreatAsAtomicUnit=on
  If Action Subsystem3 : Subsystem  TreatAsAtomicUnit=on
  If1 : If
  Merge : Merge
  Merge1 : Merge
  Zero : Constant  OutDataTypeStr=int32
  pn : Outport
  vn : Outport  Port=2
  an : Outport  Port=3
  value : Outport  Port=4
  wires:
  v/1 -> If Action Subsystem2/1(v), If/1
  bVelocityMove/1 -> If Action Subsystem/1(bVelocityMove)
  vTimer/1 -> If Action Subsystem/2(vTimer)
  vT/1 -> If Action Subsystem/3(vT)
  If1/1 -> If Action Subsystem1/Action
  a/1 -> If Action Subsystem3/1(a), If1/1
  pos_max/1 -> pn/1
  Zero/1 -> value/1
  If/1 -> If Action Subsystem/Action
  If/2 -> If Action Subsystem2/Action
  If Action Subsystem2/1(vn) -> Merge/1
  If Action Subsystem/1(vn) -> Merge/2
  Merge/1 -> vn/1
  If1/2 -> If Action Subsystem3/Action
  Merge1/1 -> an/1
  If Action Subsystem3/1(an) -> Merge1/1
  If Action Subsystem1/1(an) -> Merge1/2

== system MinimumJerkPlanner/do_step/Enabled Subsystem/If Action Subsystem1 ==
  p : Inport
  v : Inport  Port=2
  a : Inport  Port=3
  Action Port : ActionPort  ActionPortLabel=else
  Zero : Constant  Value=0  OutDataTypeStr=int32
  pn : Outport
  vn : Outport  Port=2
  an : Outport  Port=3
  value : Outport  Port=4
  wires:
  Zero/1 -> value/1
  p/1 -> pn/1
  a/1 -> an/1
  v/1 -> vn/1

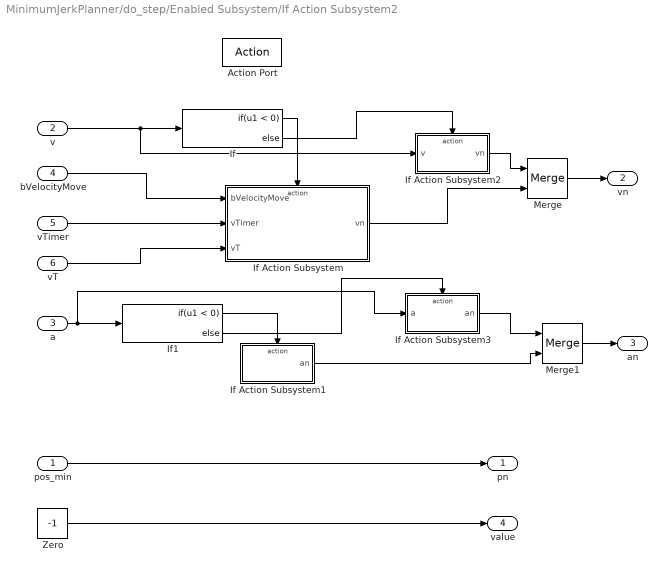
== system MinimumJerkPlanner/do_step/Enabled Subsystem/If Action Subsystem2 ==
  pos_min : Inport
  v : Inport  Port=2
  a : Inport  Port=3
  bVelocityMove : Inport  Port=4
  vTimer : Inport  Port=5
  vT : Inport  Port=6
  Action Port : ActionPort  ActionPortLabel=if(u1<=u2)
  If : If  IfExpression=u1 < 0
  If Action Subsystem : Subsystem  TreatAsAtomicUnit=on
  If Action Subsystem1 : Subsystem  TreatAsAtomicUnit=on
  If Action Subsystem2 : Subsystem  TreatAsAtomicUnit=on
  If Action Subsystem3 : Subsystem  TreatAsAtomicUnit=on
  If1 : If  IfExpression=u1 < 0
  Merge : Merge
  Merge1 : Merge
  Zero : Constant  Value=-1  OutDataTypeStr=int32
  pn : Outport
  vn : Outport  Port=2
  an : Outport  Port=3
  value : Outport  Port=4
  wires:
  pos_min/1 -> pn/1
  bVelocityMove/1 -> If Action Subsystem/1(bVelocityMove)
  a/1 -> If Action Subsystem3/1(a), If1/1
  v/1 -> If Action Subsystem2/1(v), If/1
  vT/1 -> If Action Subsystem/3(vT)
  Zero/1 -> value/1
  vTimer/1 -> If Action Subsystem/2(vTimer)
  If Action Subsystem1/1(an) -> Merge1/2
  If Action Subsystem/1(vn) -> Merge/2
  If1/1 -> If Action Subsystem1/Action
  If/1 -> If Action Subsystem/Action
  If/2 -> If Action Subsystem2/Action
  If Action Subsystem2/1(vn) -> Merge/1
  Merge/1 -> vn/1
  If1/2 -> If Action Subsystem3/Action
  If Action Subsystem3/1(an) -> Merge1/1
  Merge1/1 -> an/1

== system MinimumJerkPlanner/do_step/Enabled Subsystem/If Action Subsystem/If Action Subsystem ==
  bVelocityMove : Inport
  vTimer : Inport  Port=2
  vT : Inport  Port=3
  Action Port : ActionPort  ActionPortLabel=if(u1 > 0)
  Constant : Constant  Value=0  OutDataTypeStr=single
  If : If  IfExpression=u1 ~= 0  ShowElse=off
  If Action Subsystem : Subsystem  TreatAsAtomicUnit=on
  Less Than : RelationalOperator  Operator=<  OutDataTypeStr=boolean  RndMeth=Simplest  InputSameDT=off
  OR : Logic  Operator=OR  IconShape=distinctive  AllPortsSameDT=off  OutDataTypeStr=boolean
  vn : Outport
  wires:
  Constant/1 -> vn/1
  bVelocityMove/1 -> OR/1
  vTimer/1 -> Less Than/1
  vT/1 -> Less Than/2
  Less Than/1 -> OR/2
  OR/1 -> If/1
  If/1 -> If Action Subsystem/Action

== system MinimumJerkPlanner/do_step/Enabled Subsystem/If Action Subsystem/If Action Subsystem1 ==
  Action Port : ActionPort  ActionPortLabel=if(u1 > 0)
  Constant : Constant  Value=0  OutDataTypeStr=single
  an : Outport
  wires:
  Constant/1 -> an/1

== system MinimumJerkPlanner/do_step/Enabled Subsystem/If Action Subsystem/If Action Subsystem2 ==
  v : Inport
  Action Port : ActionPort  ActionPortLabel=else
  vn : Outport
  wires:
  v/1 -> vn/1

== system MinimumJerkPlanner/do_step/Enabled Subsystem/If Action Subsystem/If Action Subsystem3 ==
  a : Inport
  Action Port : ActionPort  ActionPortLabel=else
  an : Outport
  wires:
  a/1 -> an/1

== system MinimumJerkPlanner/do_step/Enabled Subsystem/If Action Subsystem2/If Action Subsystem ==
  bVelocityMove : Inport
  vTimer : Inport  Port=2
  vT : Inport  Port=3
  Action Port : ActionPort  ActionPortLabel=if(u1 < 0)
  Constant : Constant  Value=0  OutDataTypeStr=single
  If : If  IfExpression=u1 ~= 0  ShowElse=off
  If Action Subsystem : Subsystem  TreatAsAtomicUnit=on
  Less Than : RelationalOperator  Operator=<  OutDataTypeStr=boolean  RndMeth=Simplest  InputSameDT=off
  OR : Logic  Operator=OR  IconShape=distinctive  AllPortsSameDT=off  OutDataTypeStr=boolean
  vn : Outport
  wires:
  Constant/1 -> vn/1
  bVelocityMove/1 -> OR/1
  vTimer/1 -> Less Than/1
  vT/1 -> Less Than/2
  Less Than/1 -> OR/2
  OR/1 -> If/1
  If/1 -> If Action Subsystem/Action

== system MinimumJerkPlanner/do_step/Enabled Subsystem/If Action Subsystem2/If Action Subsystem1 ==
  Action Port : ActionPort  ActionPortLabel=if(u1 < 0)
  Constant : Constant  Value=0  OutDataTypeStr=single
  an : Outport
  wires:
  Constant/1 -> an/1

== system MinimumJerkPlanner/do_step/Enabled Subsystem/If Action Subsystem2/If Action Subsystem2 ==
  v : Inport
  Action Port : ActionPort  ActionPortLabel=else
  vn : Outport
  wires:
  v/1 -> vn/1

== system MinimumJerkPlanner/do_step/Enabled Subsystem/If Action Subsystem2/If Action Subsystem3 ==
  a : Inport
  Action Port : ActionPort  ActionPortLabel=else
  an : Outport
  wires:
  a/1 -> an/1

== system MinimumJerkPlanner/do_step/Enabled Subsystem/If Action Subsystem/If Action Subsystem/If Action Subsystem ==
  Action Port : ActionPort  ActionPortLabel=if(u1 ~= 0)
  Function Caller : FunctionCaller  FunctionPrototype=Trajectory_velocity_stop()  InputArgumentSpecifications=<Enter example>  OutputArgumentSpecifications=<Enter example>

== system MinimumJerkPlanner/do_step/Enabled Subsystem/If Action Subsystem2/If Action Subsystem/If Action Subsystem ==
  Action Port : ActionPort  ActionPortLabel=if(u1 ~= 0)
  Function Caller : FunctionCaller  FunctionPrototype=Trajectory_velocity_stop()  InputArgumentSpecifications=<Enter example>  OutputArgumentSpecifications=<Enter example>
